simulink model "dynamics_lab2_part2_alessio2"  (Simulink 8.0)
settings: Solver=ode1  StartTime=0.0  StopTime=1000  FixedStep=0.1  RelTol=1e-3
InitFcn:
  | clear all;close all;clc;warning off all;
  | 
  | 
  | 
  | mu=398600; %earth radius and universal gravitation constant
  | 
  | %Spacecraft orbit
  | R=26600; %orbit radius from center of earth
  | wo=sqrt(mu/(R)^3);
  | 
  | 
  | %Spacecraft Inertia conditions
  | Ix=480; Iy=520; Iz=420;
  | Imo=[Ix 0 0; 0 Iy 0;0 0 Iz]; %Moment of inertia matrix
  | Iinv=inv(Imo); %Moment of inertia inverse goes in dynamics block
libraries: aerospace x2
settings Model: Creator=bleonard  LastModifiedBy=Grompone
settings DataIOCC: SignalLoggingSaveFormat=ModelDataLogs
settings OptimizationCC: InitFltsAndDblsToZero=on
settings DebuggingCC: SaveWithParameterizedLinksMsg=none  MultiTaskCondExecSysMsg=none  FcnCallInpInsideContextMsg=EnableAllAsWarning  StrictBusMsg=None
settings RTWCC: IncludeERTFirstTime=on
settings GRTTargetCC: CombineOutputUpdateFcns=off  GRTInterface=on

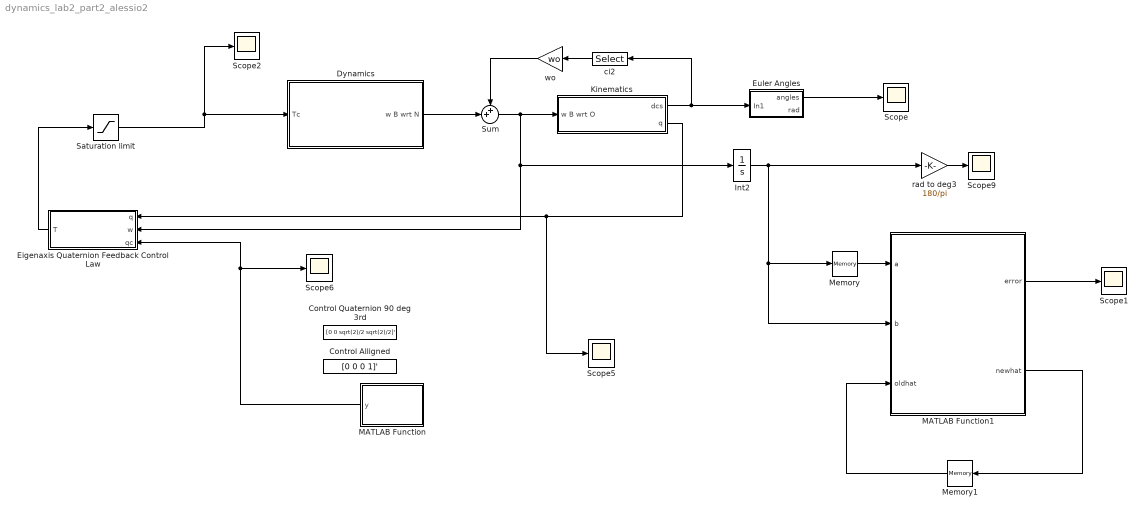
== system dynamics_lab2_part2_alessio2 ==
  Control Alligned : Constant  Value=[0 0 0 1]'
  Control Quaternion 90 deg 3rd : Constant  Value=[0 0 sqrt(2)/2 sqrt(2)/2]'
  Dynamics : Subsystem
  Eigenaxis Quaternion Feedback Control Law : Subsystem
  Euler Angles : Subsystem
  Int2 : Integrator  InitialCondition="[0  0  0]'"
  Kinematics : Subsystem
  MATLAB Function : MATLAB Function  TreatAsAtomicUnit=on
  MATLAB Function1 : MATLAB Function  TreatAsAtomicUnit=on
  Memory : Memory  X0=[0,0,0]
  Memory1 : Memory  X0=eye(3)
  Saturation limit : Saturate  UpperLimit=1.2  LowerLimit=-1.2
  Scope{,1..2,5..6,9} (6 alike) : Scope
      Scope settings: YMin=-200  YMax=200
      Scope2 settings: YMin=-0.05  YMax=0.65  SaveName=ScopeData2
      Scope5 settings: YMin=-200  YMax=200  SaveName=ScopeData5
      Scope6 settings: YMin=-200  YMax=200  SaveName=ScopeData7
      Scope9 settings: YMin=-200  YMax=200  SaveName=ScopeData10
  Sum : Sum  Inputs=++|
  ci2 : Selector  InputPortWidth=9  IndexOptions=Index vector (dialog)  Indices=[4 5 6]  OutputSizes=1
  rad to deg3 : Gain  Gain=180/pi
  wo : Gain  Gain=wo
  wires:
  Dynamics/1(w B wrt N) -> Sum/2
  Sum/1 -> Int2/1, Eigenaxis Quaternion Feedback Control Law/2(w), Kinematics/1(w B wrt O)
  Kinematics/1(dcs) -> Euler Angles/1(In1), ci2/1
  ci2/1 -> wo/1
  Euler Angles/1(angles) -> Scope/1
  Int2/1 -> rad to deg3/1, Memory/1, MATLAB Function1/2(b)
  rad to deg3/1 -> Scope9/1
  Memory/1 -> MATLAB Function1/1(a)
  MATLAB Function1/2(newhat) -> Memory1/1
  Memory1/1 -> MATLAB Function1/3(oldhat)
  MATLAB Function1/1(error) -> Scope1/1
  Eigenaxis Quaternion Feedback Control Law/1(T) -> Saturation limit/1
  Saturation limit/1 -> Scope2/1, Dynamics/1(Tc)
  MATLAB Function/1(y) -> Scope6/1, Eigenaxis Quaternion Feedback Control Law/3(qc)
  Kinematics/2(q) -> Scope5/1, Eigenaxis Quaternion Feedback Control Law/1(q)
  wo/1 -> Sum/1

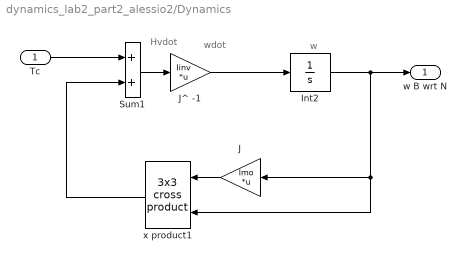
== system dynamics_lab2_part2_alessio2/Dynamics ==
  note: wdot
  note: Hvdot
  note: w
  Tc : Inport
  "   J^ -1" : Gain  Gain=Iinv  Multiplication=Matrix(K*u)  SaturateOnIntegerOverflow=on  OutDataTypeStr=Inherit: Same as input  ParamDataTypeStr=Inherit: Same as input
  Int2 : Integrator  InitialCondition=[0 0 0]'
  J : Gain  Gain=Imo  Multiplication=Matrix(K*u)  SaturateOnIntegerOverflow=on  OutDataTypeStr=Inherit: Same as input  ParamDataTypeStr=Inherit: Same as input
  Sum1 : Sum  SaturateOnIntegerOverflow=on  InputSameDT=on  OutDataTypeStr=Inherit: Same as first input
  x product1 : aerospace/Axes Transformations/3x3 cross product
  w B wrt N : Outport
  wires:
  Sum1/1 -> "   J^ -1"/1
  Int2/1 -> J/1, x product1/2, w B wrt N/1
  "   J^ -1"/1 -> Int2/1
  J/1 -> x product1/1
  Tc/1 -> Sum1/1
  x product1/1 -> Sum1/2

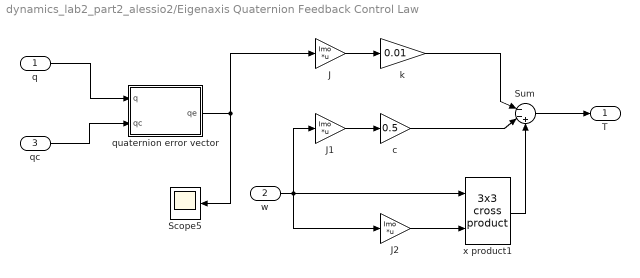
== system dynamics_lab2_part2_alessio2/Eigenaxis Quaternion Feedback Control Law ==
  q : Inport
  w : Inport  Port=2
  qc : Inport  Port=3
  J : Gain  Gain=Imo  Multiplication=Matrix(K*u)
  J1 : Gain  Gain=Imo  Multiplication=Matrix(K*u)
  J2 : Gain  Gain=Imo  Multiplication=Matrix(K*u)
  Scope5 : Scope
      settings: YMin=-200  YMax=200  SaveName=ScopeData6
  Sum : Sum  Inputs=|--+
  c : Gain  Gain=0.5
  k : Gain  Gain=0.01
  quaternion error vector : MATLAB Function  TreatAsAtomicUnit=on
  x product1 : aerospace/Axes Transformations/3x3 cross product
  T : Outport
  wires:
  J/1 -> k/1
  quaternion error vector/1(qe) -> Scope5/1, J/1
  J1/1 -> c/1
  w/1 -> J2/1, J1/1, x product1/1
  k/1 -> Sum/1
  c/1 -> Sum/2
  x product1/1 -> Sum/3
  q/1 -> quaternion error vector/1(q)
  qc/1 -> quaternion error vector/2(qc)
  J2/1 -> x product1/2
  Sum/1 -> T/1

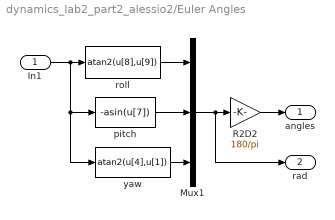
== system dynamics_lab2_part2_alessio2/Euler Angles ==
  In1 : Inport
  Mux1 : Mux  Inputs=3
  R2D2 : Gain  Gain=180/pi  SampleTime=0.1
  pitch : Fcn  Expr=-asin(u[7])
  roll : Fcn  Expr=atan2(u[8],u[9])
  yaw : Fcn  Expr=atan2(u[4],u[1])
  angles : Outport
  rad : Outport  Port=2
  wires:
  roll/1 -> Mux1/1
  yaw/1 -> Mux1/3
  pitch/1 -> Mux1/2
  Mux1/1 -> rad/1, R2D2/1
  In1/1 -> roll/1, pitch/1, yaw/1
  R2D2/1 -> angles/1

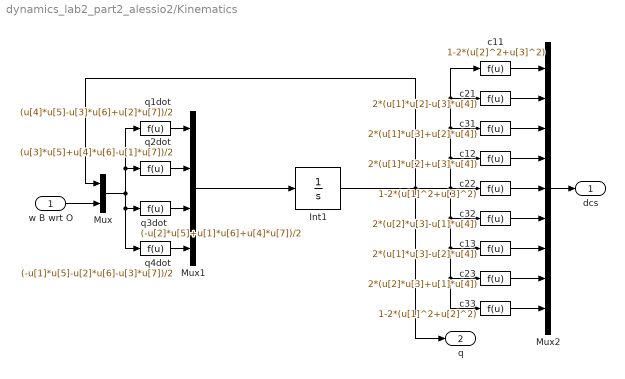
== system dynamics_lab2_part2_alessio2/Kinematics ==
  w B wrt O : Inport
  Int1 : Integrator  InitialCondition=[0 0 0 1]'
  Mux : Mux  Inputs=2
  Mux1 : Mux
  Mux2 : Mux  Inputs=9
  c11 : Fcn  Expr=1-2*(u[2]^2+u[3]^2)
  c12 : Fcn  Expr=2*(u[1]*u[2]+u[3]*u[4])
  c13 : Fcn  Expr=2*(u[1]*u[3]-u[2]*u[4])
  c21 : Fcn  Expr=2*(u[1]*u[2]-u[3]*u[4])
  c22 : Fcn  Expr=1-2*(u[1]^2+u[3]^2)
  c23 : Fcn  Expr=2*(u[2]*u[3]+u[1]*u[4])
  c31 : Fcn  Expr=2*(u[1]*u[3]+u[2]*u[4])
  c32 : Fcn  Expr=2*(u[2]*u[3]-u[1]*u[4])
  c33 : Fcn  Expr=1-2*(u[1]^2+u[2]^2)
  q1dot : Fcn  Expr=(u[4]*u[5]-u[3]*u[6]+u[2]*u[7])/2
  q2dot : Fcn  Expr=(u[3]*u[5]+u[4]*u[6]-u[1]*u[7])/2
  q3dot : Fcn  Expr=(-u[2]*u[5]+u[1]*u[6]+u[4]*u[7])/2
  q4dot : Fcn  Expr=(-u[1]*u[5]-u[2]*u[6]-u[3]*u[7])/2
  dcs : Outport
  q : Outport  Port=2
  wires:
  Mux/1 -> q4dot/1, q3dot/1, q1dot/1, q2dot/1
  q1dot/1 -> Mux1/1
  q2dot/1 -> Mux1/2
  q3dot/1 -> Mux1/3
  q4dot/1 -> Mux1/4
  Int1/1 -> Mux/1, c22/1, c11/1, c21/1, c31/1, c12/1, c32/1, c13/1, c33/1, c23/1, q/1
  c11/1 -> Mux2/1
  c22/1 -> Mux2/5
  c33/1 -> Mux2/9
  c21/1 -> Mux2/2
  c31/1 -> Mux2/3
  c12/1 -> Mux2/4
  c32/1 -> Mux2/6
  c13/1 -> Mux2/7
  c23/1 -> Mux2/8
  Mux1/1 -> Int1/1
  w B wrt O/1 -> Mux/2
  Mux2/1 -> dcs/1

== matlab function MATLAB Function1 ==
  data: a input double; b input double; oldhat input double; error output double; newhat output double
function [error,newhat] = fcn(a,b,oldhat)

e1=1/sqrt(3);
e2=1/sqrt(3);
e3=0;
e = [e1,e2,e3];

roll = b(1) - a(1);
pitch = b(2) - a(2);
yaw = b(3) - a(3);

Cba = [1, yaw, -pitch; -yaw, 1, roll; pitch, -roll, 1];

newhat = Cba*oldhat;
error = e*newhat - e*oldhat;

== matlab function MATLAB Function ==
  data: y output double
function y = fcn
%#codegen

alfa=25*pi/180;

e1=1/sqrt(3);
e2=1/sqrt(3);
e3=0;


q1=sin(alfa/2)*e1;
q2=sin(alfa/2)*e2;
q3=sin(alfa/2)*e3;
q4=cos(alfa/2);


y = [q1 q2 q3 q4];

== matlab function Eigenaxis Quaternion Feedback Control Law/quaternion error vector ==
  data: q input double; qe output double; qc input double
function qe = fcn(q,qc)
%#codegen

qcm=[qc(4) qc(3) -qc(2) -qc(1);-qc(3) qc(4) qc(1) -qc(2);qc(2) -qc(1) qc(4) -qc(3);qc(1) qc(2) qc(3) qc(4)];


qem = qcm*q; 

qe=[qem(1) qem(2) qem(3)]';
